simulink model "Status"  (R2018a)
settings: Solver=VariableStepAuto  StartTime=0.0  StopTime=10.0  RelTol=1e-3
settings Model: Creator=JITESH  LastModifiedBy=shami

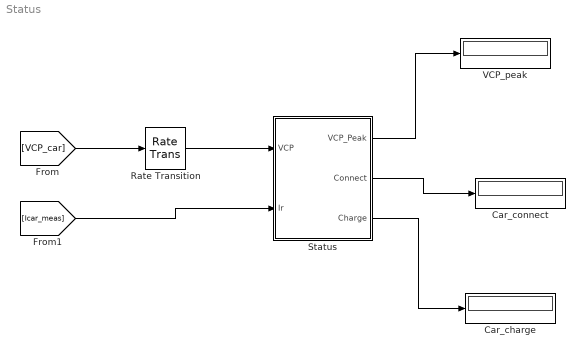
== system Status ==
  Car_charge : Display
  Car_connect : Display
  Rate Transition : RateTransition
  Status : Subsystem
  VCP_peak : Display
  wires:
  Rate Transition/1 -> Status/1(VCP)
  [VCP_car] -> Rate Transition/1
  [Icar_meas] -> Status/2(Ir)
  Status/1(VCP_Peak) -> VCP_peak/1
  Status/2("Connect ") -> Car_connect/1
  Status/3("Charge ") -> Car_charge/1

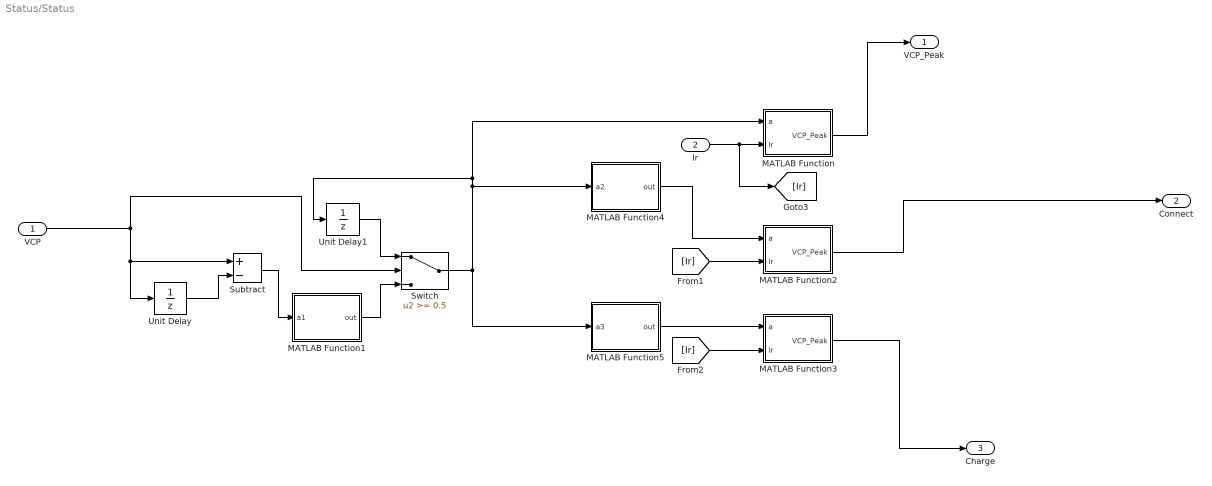
== system Status/Status ==
  VCP : Inport
  Ir : Inport  Port=2
  MATLAB Function : MATLAB Function  TreatAsAtomicUnit=on
  MATLAB Function1 : MATLAB Function  TreatAsAtomicUnit=on
  MATLAB Function2 : MATLAB Function  TreatAsAtomicUnit=on
  MATLAB Function3 : MATLAB Function  TreatAsAtomicUnit=on
  MATLAB Function4 : MATLAB Function  TreatAsAtomicUnit=on
  MATLAB Function5 : MATLAB Function  TreatAsAtomicUnit=on
  Subtract : Sum  Inputs=+-
  Switch : Switch  Threshold=0.5
  Unit Delay : UnitDelay  SampleTime=-1
  Unit Delay1 : UnitDelay  SampleTime=-1
  VCP_Peak : Outport
  "Connect " : Outport  Port=2
  "Charge " : Outport  Port=3
  wires:
  Switch/1 -> MATLAB Function5/1(a3), MATLAB Function4/1(a2), Unit Delay1/1, MATLAB Function/1(a)
  Unit Delay/1 -> Subtract/2
  Unit Delay1/1 -> Switch/1
  VCP/1 -> Switch/2, Unit Delay/1, Subtract/1
  Subtract/1 -> MATLAB Function1/1(a1)
  MATLAB Function1/1(out) -> Switch/3
  MATLAB Function4/1(out) -> MATLAB Function2/1(a)
  MATLAB Function5/1(out) -> MATLAB Function3/1(a)
  MATLAB Function/1(VCP_Peak) -> VCP_Peak/1
  MATLAB Function2/1(VCP_Peak) -> "Connect "/1
  MATLAB Function3/1(VCP_Peak) -> "Charge "/1
  Ir/1 -> MATLAB Function/2(Ir), [Ir]
  [Ir] -> MATLAB Function2/2(Ir)
  [Ir] -> MATLAB Function3/2(Ir)

== matlab function Status/MATLAB Function1 ==
  data: a1 input; out output
function out = fcn(a1)
int temp = 0;
if(a1 > 1)
    y = 1;
    int temp = y;
elseif (a1 < 1)
    y = 0;    
    int temp = y;

elseif (a1 == 1)
    y = temp;
    
end

out = y;

== matlab function Status/MATLAB Function ==
  data: a input; Ir input; VCP_Peak output
function VCP_Peak = fcn(a, Ir)
int temp = 0;
if(Ir < 1e-6)
    y = 0;
    int temp = y

elseif (Ir > 1e-6)
    y = a;    
    int temp = y;

elseif (Ir == 1e-6)
    y = temp;
end

VCP_Peak = y;

== matlab function Status/MATLAB Function2 ==
  data: a input; Ir input; VCP_Peak output
function VCP_Peak = fcn(a, Ir)
int temp = 0;
if(Ir < 1e-6)
    y = 0;
    int temp = y

elseif (Ir > 1e-6)
    y = a;    
    int temp = y;

elseif (Ir == 1e-6)
    y = temp;
end

VCP_Peak = y;

== matlab function Status/MATLAB Function3 ==
  data: a input; Ir input; VCP_Peak output
function VCP_Peak = fcn(a, Ir)
int temp = 0;
if(Ir < 1e-6)
    y = 0;
    int temp = y

elseif (Ir > 1e-6)
    y = a;    
    int temp = y;

elseif (Ir == 1e-6)
    y = temp;
end

VCP_Peak = y;

== matlab function Status/MATLAB Function4 ==
  data: a2 input; out output
function out = fcn(a2)
int temp = 0;
if(a2 < 9)
    y = 1;  
    int temp = y;
elseif (a2 > 9)
    y = 0;    
    int temp = y;
    
elseif (a2 == 9)
    y = temp;
end

out = y;

== matlab function Status/MATLAB Function5 ==
  data: a3 input; out output
function out = fcn(a3)
int temp = 0;
if(a3 < 6)
    y = 1;  
    int temp = y;
elseif(a3 > 6)
    y = 0;    
    int temp = y;
    
elseif (a3 == 6)
    y = temp;
          
end

out = y;
